simulink model "two_time_domains_synch"  (R2025b)
settings: Solver=VariableStepAuto  StartTime=0.0  StopTime=0.2  FixedStep=ts_afe  MaxStep=tc
undefined symbols (not defined in the file): fPWM_AFE, omega0, tc, time_gain_afe_module_1, time_gain_afe_module_2, time_gain_inv_module_1, time_gain_inv_module_2, trgo_th_generator, ts_afe, ts_inv
settings Model: SimulationMode=accelerator  Creator=dbagn  LastModifiedBy=dbagn
settings SolverCC: NumberNewtonIterations=3.0  ZeroCrossControl=DisableAll  AlgebraicLoopSolver=TrustRegion  SolverResetMethod=Robust
settings DataIOCC: ReturnWorkspaceOutputs=off
settings OptimizationCC: ReuseModelBlockBuffer=off
settings DebuggingCC: UnconnectedInputMsg=warning  UnconnectedOutputMsg=warning  UnconnectedLineMsg=warning
settings ModelReferenceCC: EnableRefExpFcnMdlSchedulingChecks=on
settings SFSimCC: CustomCodeUndefinedFunction=ThrowError  DefaultCustomCodeDeterministicFunctions=All
settings SFSimCC: SimCustomHeaderCode=|
  | #include "mavgflt.h"
  | #include "mavgflt_simulink.h"
  | #include "bemf_obsv.h"
  | #include "bemf_obsv_simulink.h"
  | #include "bemf_obsv_load_est.h"
  | #include "bemf_obsv_load_est_simulink.h"
  | #include "dqvector_pi.h"
  | #include "dqvector_pi_simulink.h"
  | #include "sv_pwm_simulink.h"
  | #include "sv_pwm.h"
  | #include "first_harmonic_tracker.h"
  | #include "first_harmonic_tracker_simulink.h"
  | #include "dqpll_thyr.h"
  | #include "dqpll_thyr_simulink.h"
  | #include "dqpll_grid.h"
  | #include "dqpll_grid_simulink.h"
settings SFSimCC: SimUserSources=|
  | "mavgflt_simulink.c"
  | "mavgflt.c"
  | "bemf_obsv_simulink.c"
  | "bemf_obsv.c"
  | "bemf_obsv_load_est_simulink.c"
  | "bemf_obsv_load_est.c"
  | "dqvector_pi.c"
  | "dqvector_pi_simulink.c"
  | "sv_pwm_simulink.c"
  | "sv_pwm.c"
  | "first_harmonic_tracker_simulink.c"
  | "first_harmonic_tracker.c"
  | "dqpll_thyr_simulink.c"
  | "dqpll_thyr.c"
  | "dqpll_grid_simulink.c"
  | "dqpll_grid.c"
settings SFSimCC: SimUserIncludeDirs=|
  | include
  | src
settings RTWCC: GPUComputeCapability=3.5  DLArmComputeVersion=19.05

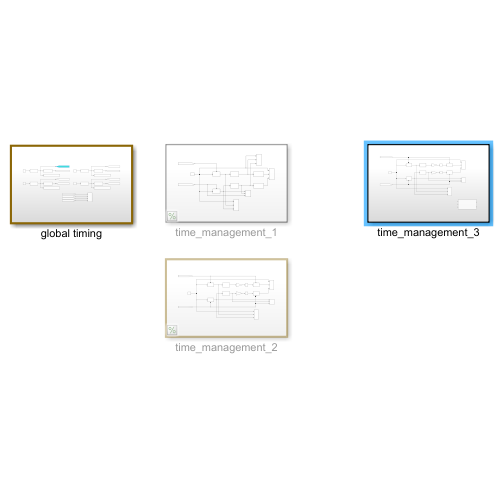
[thumbnail: Simulink's stored preview of the top-level diagram]
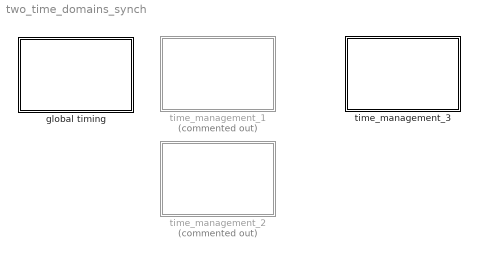
== system two_time_domains_synch ==
  global timing : Subsystem
  time_management_1 : Subsystem  Commented=on
  time_management_2 : Subsystem  Commented=on
  time_management_3 : Subsystem

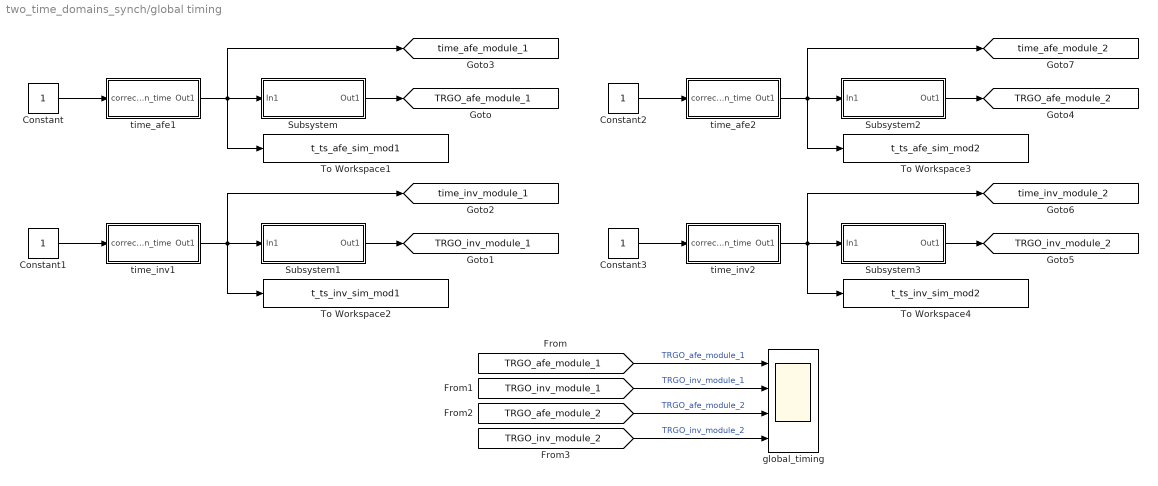
== system two_time_domains_synch/global timing ==
  Constant{,1..3} (4 alike) : Constant
  Subsystem : Subsystem  mask{samplig_time=ts_afe}
      mask prompts: samplig_time "Sampling Time"
      mask Display: disp('TRGO Generator');
  Subsystem1 : Subsystem  mask{samplig_time=ts_inv}
      mask prompts: samplig_time "Sampling Time"
      mask Display: disp('TRGO Generator');
  Subsystem2 : Subsystem  mask{samplig_time=ts_afe}
      mask prompts: samplig_time "Sampling Time"
      mask Display: disp('TRGO Generator');
  Subsystem3 : Subsystem  mask{samplig_time=ts_inv}
      mask prompts: samplig_time "Sampling Time"
      mask Display: disp('TRGO Generator');
  To Workspace1 : ToWorkspace  VariableName=t_ts_afe_sim_mod1  SampleTime=ts_afe
      settings: MaxDataPoints=Ns_afe
  To Workspace2 : ToWorkspace  VariableName=t_ts_inv_sim_mod1  SampleTime=ts_afe
      settings: MaxDataPoints=Ns_afe
  To Workspace3 : ToWorkspace  VariableName=t_ts_afe_sim_mod2  SampleTime=ts_afe
      settings: MaxDataPoints=Ns_afe
  To Workspace4 : ToWorkspace  VariableName=t_ts_inv_sim_mod2  SampleTime=ts_afe
      settings: MaxDataPoints=Ns_afe
  global_timing : Scope  NumInputPorts=4
      settings: SampleTime=tc  ActiveDisplayYMinimum=-0.125  ActiveDisplayYMaximum=1.125
  time_afe1 : Subsystem  mask{k=time_gain_afe_module_1}
      mask prompts: k "Time Gain"
      mask Display:
      | disp('time-gen');
      | port_label('input', 1, 'crt');
      | port_label('output', 1, 'tout');
  time_afe2 : Subsystem  mask{k=time_gain_afe_module_2}
      mask prompts: k "Time Gain"
      mask Display:
      | disp('time-gen');
      | port_label('input', 1, 'crt');
      | port_label('output', 1, 'tout');
  time_inv1 : Subsystem  mask{k=time_gain_inv_module_1}
      mask prompts: k "Time Gain"
      mask Display:
      | disp('time-gen');
      | port_label('input', 1, 'crt');
      | port_label('output', 1, 'tout');
  time_inv2 : Subsystem  mask{k=time_gain_inv_module_2}
      mask prompts: k "Time Gain"
      mask Display:
      | disp('time-gen');
      | port_label('input', 1, 'crt');
      | port_label('output', 1, 'tout');
  tag scope: TRGO_afe_module_1=global, TRGO_afe_module_2=global, TRGO_inv_module_1=global, TRGO_inv_module_2=global, time_afe_module_1=global, time_afe_module_2=global, time_inv_module_1=global, time_inv_module_2=global
  wires:
  Constant/1 -> time_afe1/1(correction_time)
  time_afe1/1(Out1) -> To Workspace1/1, [time_afe_module_1], Subsystem/1(In1)
  Subsystem/1(Out1) -> [TRGO_afe_module_1]
  Subsystem1/1(Out1) -> [TRGO_inv_module_1]
  time_inv1/1(Out1) -> To Workspace2/1, Subsystem1/1(In1), [time_inv_module_1]
  Constant1/1 -> time_inv1/1(correction_time)
  Constant3/1 -> time_inv2/1(correction_time)
  time_inv2/1(Out1) -> [time_inv_module_2], Subsystem3/1(In1), To Workspace4/1
  Subsystem3/1(Out1) -> [TRGO_inv_module_2]
  Subsystem2/1(Out1) -> [TRGO_afe_module_2]
  time_afe2/1(Out1) -> Subsystem2/1(In1), [time_afe_module_2], To Workspace3/1
  Constant2/1 -> time_afe2/1(correction_time)
  [TRGO_inv_module_1] -> global_timing/2  "TRGO_inv_module_1"
  [TRGO_afe_module_1] -> global_timing/1  "TRGO_afe_module_1"
  [TRGO_afe_module_2] -> global_timing/3  "TRGO_afe_module_2"
  [TRGO_inv_module_2] -> global_timing/4  "TRGO_inv_module_2"

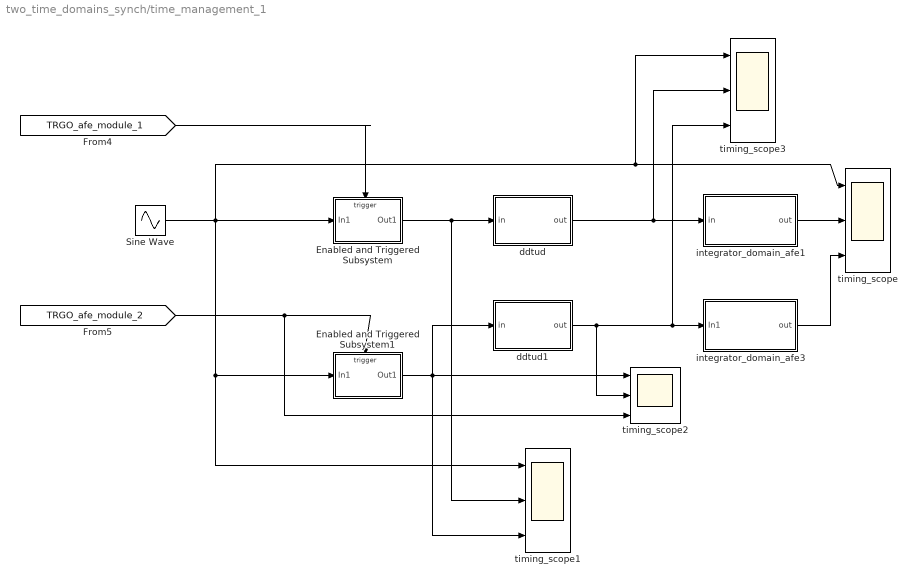
== system two_time_domains_synch/time_management_1 ==
  Enabled and Triggered Subsystem : Subsystem  TreatAsAtomicUnit=on
  Enabled and Triggered Subsystem1 : Subsystem  TreatAsAtomicUnit=on
  Sine Wave : Sin  Frequency=omega0  SampleTime=0
  ddtud : Subsystem  mask{ts=ts_afe}
      mask Display: disp('ddtud');
  ddtud1 : Subsystem  mask{ts=ts_afe %ts_afe*time_gain_afe_module_2}
      mask Display: disp('ddtud');
  integrator_domain_afe1 : Subsystem
  integrator_domain_afe3 : Subsystem
  timing_scope{,1..3} (4 alike) : Scope  NumInputPorts=3
      timing_scope settings: ActiveDisplayYMinimum=-1.25  ActiveDisplayYMaximum=1.25
      timing_scope1 settings: ActiveDisplayYMinimum=0.727291325695581  ActiveDisplayYMaximum=1.0853109656301145  DataLoggingVariableName=ScopeData2
      timing_scope2 settings: ActiveDisplayYMinimum=-1.2498314063079958  ActiveDisplayYMaximum=1.2499416649584139  DataLoggingVariableName=ScopeData3
      timing_scope3 settings: ActiveDisplayYMinimum=0.39524922118380057  ActiveDisplayYMaximum=0.65809968847352029  DataLoggingVariableName=ScopeData4
  wires:
  Sine Wave/1 -> timing_scope3/1, timing_scope/1, Enabled and Triggered Subsystem1/1(In1), timing_scope1/1, Enabled and Triggered Subsystem/1(In1)
  integrator_domain_afe1/1(out) -> timing_scope/2
  ddtud1/1(out) -> timing_scope2/2, timing_scope3/3, integrator_domain_afe3/1(In1)
  Enabled and Triggered Subsystem1/1(Out1) -> ddtud1/1(in), timing_scope1/3, timing_scope2/1
  Enabled and Triggered Subsystem/1(Out1) -> timing_scope1/2, ddtud/1(in)
  [TRGO_afe_module_2] -> Enabled and Triggered Subsystem1/Trigger, timing_scope2/3
  ddtud/1(out) -> timing_scope3/2, integrator_domain_afe1/1(in)
  [TRGO_afe_module_1] -> Enabled and Triggered Subsystem/Trigger
  integrator_domain_afe3/1(out) -> timing_scope/3

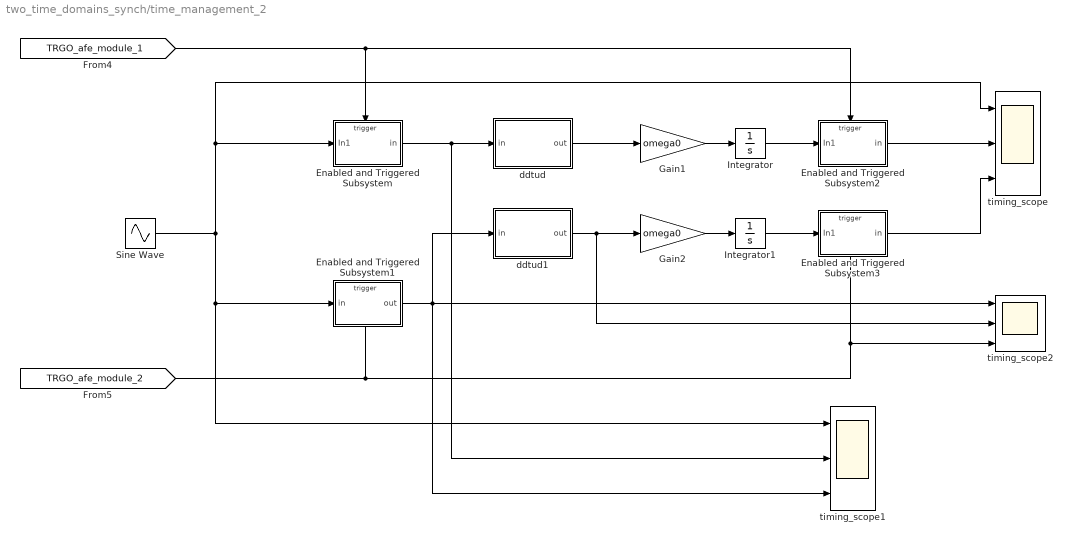
== system two_time_domains_synch/time_management_2 ==
  Enabled and Triggered Subsystem : Subsystem  TreatAsAtomicUnit=on
  Enabled and Triggered Subsystem1 : Subsystem  TreatAsAtomicUnit=on
  Enabled and Triggered Subsystem2 : Subsystem  TreatAsAtomicUnit=on
  Enabled and Triggered Subsystem3 : Subsystem  TreatAsAtomicUnit=on
  Gain1 : Gain  Gain=omega0
  Gain2 : Gain  Gain=omega0
  Integrator : Integrator
  Integrator1 : Integrator
  Sine Wave : Sin  Frequency=omega0  SampleTime=0
  ddtud : Subsystem  mask{ts=ts_afe}
      mask Display: disp('ddtud');
  ddtud1 : Subsystem  mask{ts=ts_afe}
      mask Display: disp('ddtud');
  timing_scope : Scope  NumInputPorts=3
      settings: ActiveDisplayYMinimum=0.95537901830999794  ActiveDisplayYMaximum=2.0845041307852008
  timing_scope1 : Scope  NumInputPorts=3
      settings: ActiveDisplayYMinimum=0.727291325695581  ActiveDisplayYMaximum=1.0853109656301145  DataLoggingVariableName=ScopeData2
  timing_scope2 : Scope  NumInputPorts=3
      settings: ActiveDisplayYMinimum=-1.25  ActiveDisplayYMaximum=1.25  DataLoggingVariableName=ScopeData3
  wires:
  [TRGO_afe_module_1] -> Enabled and Triggered Subsystem2/Trigger, Enabled and Triggered Subsystem/Trigger
  Enabled and Triggered Subsystem/1(in) -> ddtud/1(in), timing_scope1/2
  [TRGO_afe_module_2] -> Enabled and Triggered Subsystem1/Trigger, Enabled and Triggered Subsystem3/Trigger, timing_scope2/3
  Enabled and Triggered Subsystem1/1(out) -> timing_scope1/3, timing_scope2/1, ddtud1/1(in)
  Sine Wave/1 -> Enabled and Triggered Subsystem/1(In1), timing_scope/1, timing_scope1/1, Enabled and Triggered Subsystem1/1(in)
  ddtud1/1(out) -> Gain2/1, timing_scope2/2
  Enabled and Triggered Subsystem3/1(in) -> timing_scope/3
  Enabled and Triggered Subsystem2/1(in) -> timing_scope/2
  ddtud/1(out) -> Gain1/1
  Gain1/1 -> Integrator/1
  Integrator/1 -> Enabled and Triggered Subsystem2/1(In1)
  Gain2/1 -> Integrator1/1
  Integrator1/1 -> Enabled and Triggered Subsystem3/1(In1)

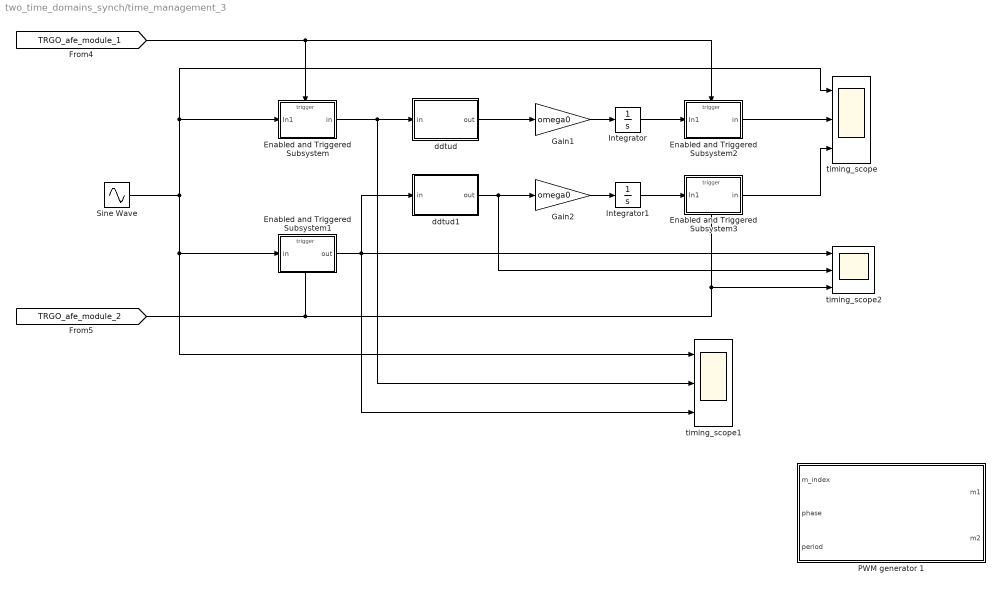
== system two_time_domains_synch/time_management_3 ==
  Enabled and Triggered Subsystem : Subsystem  TreatAsAtomicUnit=on
  Enabled and Triggered Subsystem1 : Subsystem  TreatAsAtomicUnit=on
  Enabled and Triggered Subsystem2 : Subsystem  TreatAsAtomicUnit=on
  Enabled and Triggered Subsystem3 : Subsystem  TreatAsAtomicUnit=on
  Gain1 : Gain  Gain=omega0
  Gain2 : Gain  Gain=omega0
  Integrator : Integrator
  Integrator1 : Integrator
  PWM generator 1 : Subsystem  mask{f=fPWM_AFE, m_up=1, m_low=0, dead_time=0, pos_cmd_gate=15, neg_cmd_gate=-10, polarity=1}
      mask prompts: f "Frequency (Hz)"; m_up "Max Input Modulation Value"; m_low "Min Input Modulation Value"; dead_time "Dead Time (s)"; pos_cmd_gate "Positive Gate Voltage (V)"; neg_cmd_gate "Negative Gate Voltage (V)"; polarity "Polarity (pu)"
  Sine Wave : Sin  Frequency=omega0  SampleTime=0
  ddtud : Subsystem  mask{ts=ts_afe}
      mask Display: disp('ddtud');
  ddtud1 : Subsystem  mask{ts=ts_afe}
      mask Display: disp('ddtud');
  timing_scope : Scope  NumInputPorts=3
      settings: ActiveDisplayYMinimum=0.95537901830999794  ActiveDisplayYMaximum=2.0845041307852008
  timing_scope1 : Scope  NumInputPorts=3
      settings: ActiveDisplayYMinimum=0.727291325695581  ActiveDisplayYMaximum=1.0853109656301145  DataLoggingVariableName=ScopeData2
  timing_scope2 : Scope  NumInputPorts=3
      settings: ActiveDisplayYMinimum=-1.25  ActiveDisplayYMaximum=1.25  DataLoggingVariableName=ScopeData3
  wires:
  Integrator1/1 -> Enabled and Triggered Subsystem3/1(In1)
  Gain2/1 -> Integrator1/1
  Integrator/1 -> Enabled and Triggered Subsystem2/1(In1)
  Gain1/1 -> Integrator/1
  ddtud/1(out) -> Gain1/1
  Enabled and Triggered Subsystem2/1(in) -> timing_scope/2
  Enabled and Triggered Subsystem3/1(in) -> timing_scope/3
  ddtud1/1(out) -> timing_scope2/2, Gain2/1
  Sine Wave/1 -> Enabled and Triggered Subsystem1/1(in), timing_scope1/1, timing_scope/1, Enabled and Triggered Subsystem/1(In1)
  Enabled and Triggered Subsystem1/1(out) -> ddtud1/1(in), timing_scope2/1, timing_scope1/3
  [TRGO_afe_module_2] -> timing_scope2/3, Enabled and Triggered Subsystem3/Trigger, Enabled and Triggered Subsystem1/Trigger
  Enabled and Triggered Subsystem/1(in) -> timing_scope1/2, ddtud/1(in)
  [TRGO_afe_module_1] -> Enabled and Triggered Subsystem/Trigger, Enabled and Triggered Subsystem2/Trigger

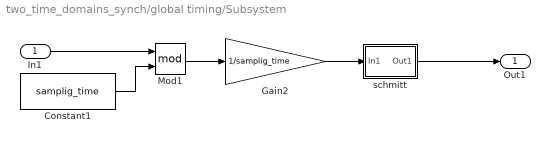
== system two_time_domains_synch/global timing/Subsystem ==
  In1 : Inport
  Constant1 : Constant  Value=samplig_time
  Gain2 : Gain  Gain=1/samplig_time
  Mod1 : Math  Operator=mod
  schmitt : Subsystem
  Out1 : Outport
  wires:
  Constant1/1 -> Mod1/2
  In1/1 -> Mod1/1
  Mod1/1 -> Gain2/1
  schmitt/1(Out1) -> Out1/1
  Gain2/1 -> schmitt/1(In1)

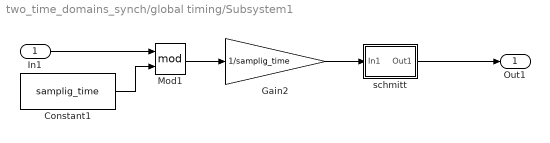
== system two_time_domains_synch/global timing/Subsystem1 ==
  In1 : Inport
  Constant1 : Constant  Value=samplig_time
  Gain2 : Gain  Gain=1/samplig_time
  Mod1 : Math  Operator=mod
  schmitt : Subsystem
  Out1 : Outport
  wires:
  Gain2/1 -> schmitt/1(In1)
  schmitt/1(Out1) -> Out1/1
  Mod1/1 -> Gain2/1
  In1/1 -> Mod1/1
  Constant1/1 -> Mod1/2

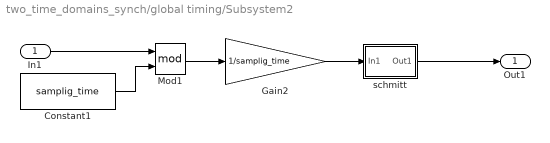
== system two_time_domains_synch/global timing/Subsystem2 ==
  In1 : Inport
  Constant1 : Constant  Value=samplig_time
  Gain2 : Gain  Gain=1/samplig_time
  Mod1 : Math  Operator=mod
  schmitt : Subsystem
  Out1 : Outport
  wires:
  Gain2/1 -> schmitt/1(In1)
  schmitt/1(Out1) -> Out1/1
  Mod1/1 -> Gain2/1
  In1/1 -> Mod1/1
  Constant1/1 -> Mod1/2

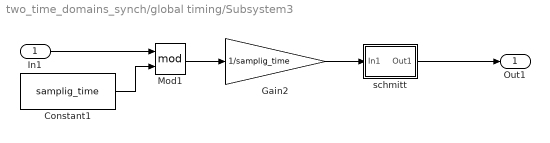
== system two_time_domains_synch/global timing/Subsystem3 ==
  In1 : Inport
  Constant1 : Constant  Value=samplig_time
  Gain2 : Gain  Gain=1/samplig_time
  Mod1 : Math  Operator=mod
  schmitt : Subsystem
  Out1 : Outport
  wires:
  Constant1/1 -> Mod1/2
  In1/1 -> Mod1/1
  Mod1/1 -> Gain2/1
  schmitt/1(Out1) -> Out1/1
  Gain2/1 -> schmitt/1(In1)

== system two_time_domains_synch/global timing/time_afe1 ==
  correction_time : Inport
  Gain : Gain  Gain=k
  Product : Product
  time_1 : Clock
  Out1 : Outport
  wires:
  time_1/1 -> Gain/1
  Gain/1 -> Product/2
  Product/1 -> Out1/1
  correction_time/1 -> Product/1

== system two_time_domains_synch/global timing/time_afe2 ==
  correction_time : Inport
  Gain : Gain  Gain=k
  Product : Product
  time_1 : Clock
  Out1 : Outport
  wires:
  correction_time/1 -> Product/1
  Product/1 -> Out1/1
  Gain/1 -> Product/2
  time_1/1 -> Gain/1

== system two_time_domains_synch/global timing/time_inv1 ==
  correction_time : Inport
  Gain : Gain  Gain=k
  Product : Product
  time_1 : Clock
  Out1 : Outport
  wires:
  correction_time/1 -> Product/1
  Product/1 -> Out1/1
  Gain/1 -> Product/2
  time_1/1 -> Gain/1

== system two_time_domains_synch/global timing/time_inv2 ==
  correction_time : Inport
  Gain : Gain  Gain=k
  Product : Product
  time_1 : Clock
  Out1 : Outport
  wires:
  time_1/1 -> Gain/1
  Gain/1 -> Product/2
  Product/1 -> Out1/1
  correction_time/1 -> Product/1

== system two_time_domains_synch/time_management_1/Enabled and Triggered Subsystem ==
  In1 : Inport
  Trigger : TriggerPort  VariantControl=(inherit)
  Out1 : Outport
  wires:
  In1/1 -> Out1/1

== system two_time_domains_synch/time_management_1/Enabled and Triggered Subsystem1 ==
  In1 : Inport
  Trigger : TriggerPort  VariantControl=(inherit)
  Out1 : Outport
  wires:
  In1/1 -> Out1/1

== system two_time_domains_synch/time_management_1/ddtud ==
  in : Inport
  Constant : Constant  Value=ts
  Propagation Delay : PropagationDelay  RunAtFixedTimeIntervals=on  SampleTime=tc
  out : Outport
  wires:
  Constant/1 -> Propagation Delay/2
  in/1 -> Propagation Delay/1
  Propagation Delay/1 -> out/1

== system two_time_domains_synch/time_management_1/ddtud1 ==
  in : Inport
  Constant : Constant  Value=ts
  Propagation Delay : PropagationDelay  RunAtFixedTimeIntervals=on  SampleTime=tc
  out : Outport
  wires:
  Propagation Delay/1 -> out/1
  in/1 -> Propagation Delay/1
  Constant/1 -> Propagation Delay/2

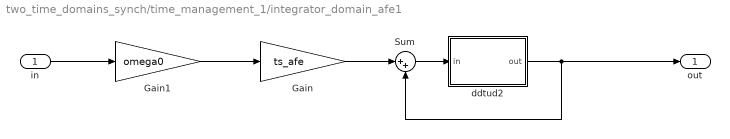
== system two_time_domains_synch/time_management_1/integrator_domain_afe1 ==
  in : Inport
  Gain : Gain  Gain=ts_afe
  Gain1 : Gain  Gain=omega0
  Sum : Sum  Inputs=|++
  ddtud2 : Subsystem  mask{ts=ts_afe}
      mask Display: disp('ddtud');
  out : Outport
  wires:
  Sum/1 -> ddtud2/1(in)
  ddtud2/1(out) -> out/1, Sum/2
  Gain/1 -> Sum/1
  in/1 -> Gain1/1
  Gain1/1 -> Gain/1

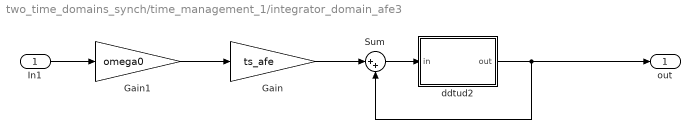
== system two_time_domains_synch/time_management_1/integrator_domain_afe3 ==
  In1 : Inport
  Gain : Gain  Gain=ts_afe
  Gain1 : Gain  Gain=omega0
  Sum : Sum  Inputs=|++
  ddtud2 : Subsystem  mask{ts=ts_afe}
      mask Display: disp('ddtud');
  out : Outport
  wires:
  In1/1 -> Gain1/1
  Gain/1 -> Sum/1
  ddtud2/1(out) -> Sum/2, out/1
  Sum/1 -> ddtud2/1(in)
  Gain1/1 -> Gain/1

== system two_time_domains_synch/time_management_2/Enabled and Triggered Subsystem ==
  In1 : Inport
  Trigger : TriggerPort  VariantControl=(inherit)
  in : Outport
  wires:
  In1/1 -> in/1

== system two_time_domains_synch/time_management_2/Enabled and Triggered Subsystem1 ==
  in : Inport
  Trigger : TriggerPort  VariantControl=(inherit)
  out : Outport
  wires:
  in/1 -> out/1

== system two_time_domains_synch/time_management_2/Enabled and Triggered Subsystem2 ==
  In1 : Inport
  Trigger : TriggerPort  VariantControl=(inherit)
  in : Outport
  wires:
  In1/1 -> in/1

== system two_time_domains_synch/time_management_2/Enabled and Triggered Subsystem3 ==
  In1 : Inport
  Trigger : TriggerPort  VariantControl=(inherit)  OutputDataType=double
  in : Outport
  wires:
  In1/1 -> in/1

== system two_time_domains_synch/time_management_2/ddtud ==
  in : Inport
  Constant : Constant  Value=ts
  Propagation Delay : PropagationDelay  SampleTime=tc
  out : Outport
  wires:
  Constant/1 -> Propagation Delay/2
  in/1 -> Propagation Delay/1
  Propagation Delay/1 -> out/1

== system two_time_domains_synch/time_management_2/ddtud1 ==
  in : Inport
  Constant : Constant  Value=ts
  Propagation Delay : PropagationDelay  SampleTime=tc
  out : Outport
  wires:
  Propagation Delay/1 -> out/1
  in/1 -> Propagation Delay/1
  Constant/1 -> Propagation Delay/2

== system two_time_domains_synch/time_management_3/Enabled and Triggered Subsystem ==
  In1 : Inport
  Trigger : TriggerPort  VariantControl=(inherit)
  in : Outport
  wires:
  In1/1 -> in/1

== system two_time_domains_synch/time_management_3/Enabled and Triggered Subsystem1 ==
  in : Inport
  Trigger : TriggerPort  VariantControl=(inherit)
  out : Outport
  wires:
  in/1 -> out/1

== system two_time_domains_synch/time_management_3/Enabled and Triggered Subsystem2 ==
  In1 : Inport
  Trigger : TriggerPort  VariantControl=(inherit)
  in : Outport
  wires:
  In1/1 -> in/1

== system two_time_domains_synch/time_management_3/Enabled and Triggered Subsystem3 ==
  In1 : Inport
  Trigger : TriggerPort  VariantControl=(inherit)  OutputDataType=double
  in : Outport
  wires:
  In1/1 -> in/1

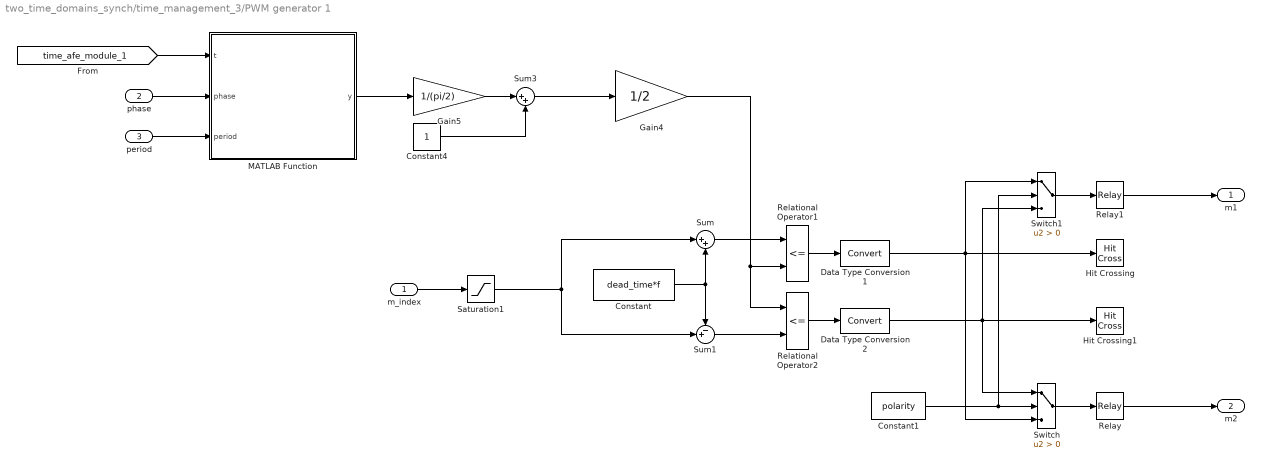
== system two_time_domains_synch/time_management_3/PWM generator 1 ==
  m_index : Inport
  phase : Inport  Port=2
  period : Inport  Port=3
  Constant : Constant  Value=dead_time*f
  Constant1 : Constant  Value=polarity
  Constant4 : Constant
  Data Type Conversion1 : DataTypeConversion
  Data Type Conversion2 : DataTypeConversion
  Gain4 : Gain  Gain=1/2
  Gain5 : Gain  Gain=1/(pi/2)
  Hit Crossing : HitCross  ShowOutputPort=off
  Hit Crossing1 : HitCross  ShowOutputPort=off
  MATLAB Function : MATLAB Function  TreatAsAtomicUnit=on
  Relational Operator1 : RelationalOperator  Operator=<=  InputSameDT=off
  Relational Operator2 : RelationalOperator  Operator=<=  InputSameDT=off
  Relay : Relay  OnOutputValue=pos_cmd_gate  OffOutputValue=neg_cmd_gate
  Relay1 : Relay  OnOutputValue=pos_cmd_gate  OffOutputValue=neg_cmd_gate
  Saturation1 : Saturate  UpperLimit=m_up  LowerLimit=m_low
  Sum : Sum  Inputs=|++  SaturateOnIntegerOverflow=on
  Sum1 : Sum  Inputs=-+|  SaturateOnIntegerOverflow=on
  Sum3 : Sum  Inputs=|++
  Switch : Switch  Criteria=u2 > Threshold  SaturateOnIntegerOverflow=off  InputSameDT=off
  Switch1 : Switch  Criteria=u2 > Threshold  SaturateOnIntegerOverflow=off  InputSameDT=off
  m1 : Outport
  m2 : Outport  Port=2
  wires:
  Relational Operator1/1 -> Data Type Conversion1/1
  m_index/1 -> Saturation1/1
  Relational Operator2/1 -> Data Type Conversion2/1
  Data Type Conversion2/1 -> Switch/1, Switch1/3, Hit Crossing1/1
  Constant/1 -> Sum/2, Sum1/1
  Saturation1/1 -> Sum/1, Sum1/2
  Sum/1 -> Relational Operator1/1
  Sum1/1 -> Relational Operator2/2
  Gain4/1 -> Relational Operator2/1, Relational Operator1/2
  Data Type Conversion1/1 -> Hit Crossing/1, Switch/3, Switch1/1
  Switch/1 -> Relay/1
  period/1 -> MATLAB Function/3(period)
  phase/1 -> MATLAB Function/2(phase)
  MATLAB Function/1(y) -> Gain5/1
  Gain5/1 -> Sum3/1
  Sum3/1 -> Gain4/1
  Constant4/1 -> Sum3/2
  Relay/1 -> m2/1
  Constant1/1 -> Switch1/2, Switch/2
  Switch1/1 -> Relay1/1
  Relay1/1 -> m1/1
  [time_afe_module_1] -> MATLAB Function/1(t)

== system two_time_domains_synch/time_management_3/ddtud ==
  in : Inport
  Constant : Constant  Value=ts
  Propagation Delay : PropagationDelay  SampleTime=tc
  out : Outport
  wires:
  Propagation Delay/1 -> out/1
  in/1 -> Propagation Delay/1
  Constant/1 -> Propagation Delay/2

== system two_time_domains_synch/time_management_3/ddtud1 ==
  in : Inport
  Constant : Constant  Value=ts
  Propagation Delay : PropagationDelay  SampleTime=tc
  out : Outport
  wires:
  Constant/1 -> Propagation Delay/2
  in/1 -> Propagation Delay/1
  Propagation Delay/1 -> out/1

== system two_time_domains_synch/global timing/Subsystem/schmitt ==
  In1 : Inport
  Constant2 : Constant
  Constant3 : Constant  Value=0
  Switch : Switch  Threshold=trgo_th_generator  SaturateOnIntegerOverflow=off  InputSameDT=off
  Out1 : Outport
  wires:
  Constant2/1 -> Switch/3
  Constant3/1 -> Switch/1
  In1/1 -> Switch/2
  Switch/1 -> Out1/1

== system two_time_domains_synch/global timing/Subsystem1/schmitt ==
  In1 : Inport
  Constant2 : Constant
  Constant3 : Constant  Value=0
  Switch : Switch  Threshold=trgo_th_generator  SaturateOnIntegerOverflow=off  InputSameDT=off
  Out1 : Outport
  wires:
  Switch/1 -> Out1/1
  In1/1 -> Switch/2
  Constant3/1 -> Switch/1
  Constant2/1 -> Switch/3

== system two_time_domains_synch/global timing/Subsystem2/schmitt ==
  In1 : Inport
  Constant2 : Constant
  Constant3 : Constant  Value=0
  Switch : Switch  Threshold=trgo_th_generator  SaturateOnIntegerOverflow=off  InputSameDT=off
  Out1 : Outport
  wires:
  Switch/1 -> Out1/1
  In1/1 -> Switch/2
  Constant3/1 -> Switch/1
  Constant2/1 -> Switch/3

== system two_time_domains_synch/global timing/Subsystem3/schmitt ==
  In1 : Inport
  Constant2 : Constant
  Constant3 : Constant  Value=0
  Switch : Switch  Threshold=trgo_th_generator  SaturateOnIntegerOverflow=off  InputSameDT=off
  Out1 : Outport
  wires:
  Constant2/1 -> Switch/3
  Constant3/1 -> Switch/1
  In1/1 -> Switch/2
  Switch/1 -> Out1/1

== system two_time_domains_synch/time_management_1/integrator_domain_afe1/ddtud2 ==
  in : Inport
  Constant : Constant  Value=ts
  Propagation Delay : PropagationDelay  RunAtFixedTimeIntervals=on  SampleTime=tc
  out : Outport
  wires:
  Propagation Delay/1 -> out/1
  in/1 -> Propagation Delay/1
  Constant/1 -> Propagation Delay/2

== system two_time_domains_synch/time_management_1/integrator_domain_afe3/ddtud2 ==
  in : Inport
  Constant : Constant  Value=ts
  Propagation Delay : PropagationDelay  RunAtFixedTimeIntervals=on  SampleTime=tc
  out : Outport
  wires:
  Constant/1 -> Propagation Delay/2
  in/1 -> Propagation Delay/1
  Propagation Delay/1 -> out/1

== matlab function two_time_domains_synch/time_management_3/PWM generator 1/MATLAB Function ==
  data: t input; y output; phase input; period input
function y = trgo(t,phase,period)
x = sin(2*pi/period*t - phase -pi/2);
y = asin(x);
